simulink model "projekt1_9_1"  (R2016b)
settings: Solver=VariableStepAuto  StartTime=0.0  StopTime=10.0  RelTol=1e-3
values from neighbouring files (symbols this model uses):
  a1 = 0.56    [projekt1.m]    (also in projekt1_5.m)
  a2 = -0.8    [projekt1.m]    (also in projekt1_5.m)
  a3 = 0.35    [projekt1.m]    (also in projekt1_5.m)
  a4 = 0.2    [projekt1.m]    (also in projekt1_5.m)
settings Model: Creator=m  LastModifiedBy=m

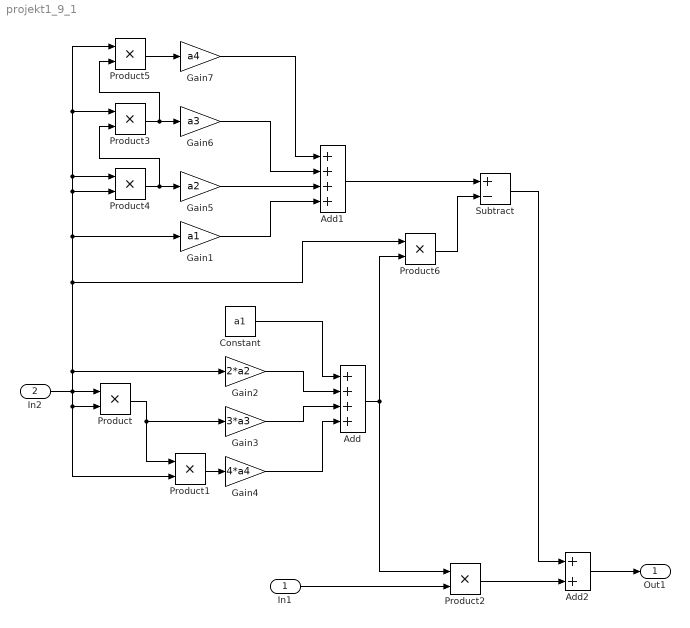
== system projekt1_9_1 ==
  In1 : Inport
  In2 : Inport  Port=2
  Add : Sum  Inputs=++++
  Add1 : Sum  Inputs=++++
  Add2 : Sum
  Constant : Constant  Value=a1
  Gain1 : Gain  Gain=a1
  Gain2 : Gain  Gain=2*a2
  Gain3 : Gain  Gain=3*a3
  Gain4 : Gain  Gain=4*a4
  Gain5 : Gain  Gain=a2
  Gain6 : Gain  Gain=a3
  Gain7 : Gain  Gain=a4
  Product{,1..6} (7 alike) : Product
  Subtract : Sum  Inputs=+-
  Out1 : Outport
  wires:
  Gain2/1 -> Add/2
  Constant/1 -> Add/1
  Gain3/1 -> Add/3
  Gain4/1 -> Add/4
  In2/1 -> Product1/2, Product/2, Product/1, Product6/1, Product5/1, Product3/1, Product4/1, Product4/2, Gain1/1, Gain2/1
  Product/1 -> Gain3/1, Product1/1
  Product1/1 -> Gain4/1
  In1/1 -> Product2/2
  Add/1 -> Product6/2, Product2/1
  Product4/1 -> Gain5/1, Product3/2
  Product3/1 -> Gain6/1, Product5/2
  Product5/1 -> Gain7/1
  Gain5/1 -> Add1/3
  Gain6/1 -> Add1/2
  Gain7/1 -> Add1/1
  Gain1/1 -> Add1/4
  Add1/1 -> Subtract/1
  Product6/1 -> Subtract/2
  Product2/1 -> Add2/2
  Subtract/1 -> Add2/1
  Add2/1 -> Out1/1
